simulink model "Lab4"  (R2023a)
settings: Solver=VariableStepAuto  StartTime=0.0  StopTime=20  RelTol=1e-3
settings Model: Creator=Lenovo  LastModifiedBy=Lenovo

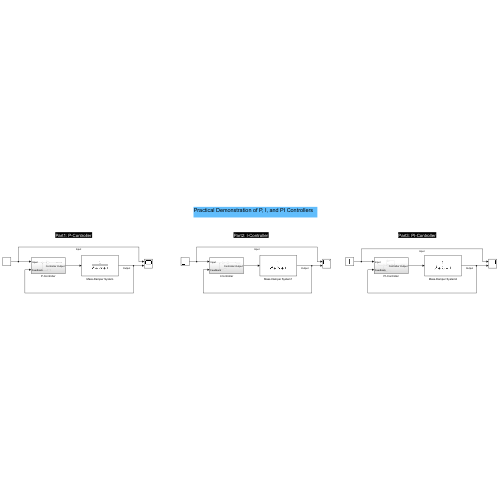
[thumbnail: Simulink's stored preview of the top-level diagram]
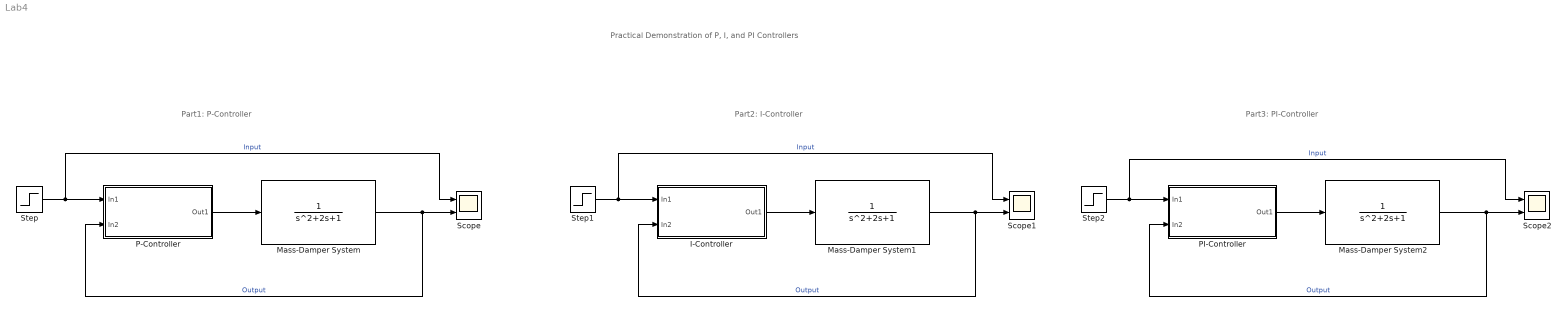
== system Lab4 ==
  note: Practical Demonstration of P, I, and PI Controllers
  note: Part1: P-Controller
  note: Part2: I-Controller
  note: Part3: PI-Controller
  I-Controller : Subsystem
  Mass-Damper System : TransferFcn
  Mass-Damper System1 : TransferFcn
  Mass-Damper System2 : TransferFcn
  P-Controller : Subsystem
  PI-Controller : Subsystem
  Scope : Scope  NumInputPorts=2
  Scope1 : Scope  NumInputPorts=2
  Scope2 : Scope  NumInputPorts=2
  Step : Step  SampleTime=0
  Step1 : Step  SampleTime=0
  Step2 : Step  SampleTime=0
  wires:
  Mass-Damper System/1 -> P-Controller/2(In2), Scope/2  "Output"
  Step/1 -> Scope/1, P-Controller/1(In1)  "Input"
  P-Controller/1(Out1) -> Mass-Damper System/1
  Mass-Damper System1/1 -> I-Controller/2(In2), Scope1/2  "Output"
  I-Controller/1(Out1) -> Mass-Damper System1/1
  Step1/1 -> Scope1/1, I-Controller/1(In1)  "Input"
  Step2/1 -> Scope2/1, PI-Controller/1(In1)  "Input"
  PI-Controller/1(Out1) -> Mass-Damper System2/1
  Mass-Damper System2/1 -> PI-Controller/2(In2), Scope2/2  "Output"

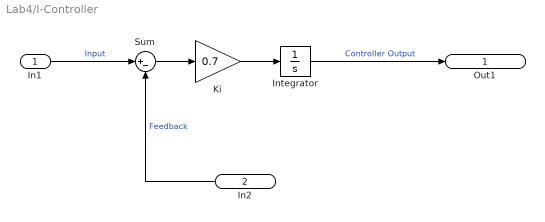
== system Lab4/I-Controller ==
  In1 : Inport
  In2 : Inport  Port=2
  Integrator : Integrator
  Ki : Gain  Gain=0.7
  Sum : Sum  Inputs=|+-
  Out1 : Outport
  wires:
  In1/1 -> Sum/1  "Input"
  Sum/1 -> Ki/1
  Ki/1 -> Integrator/1
  In2/1 -> Sum/2  "Feedback"
  Integrator/1 -> Out1/1  "Controller Output"

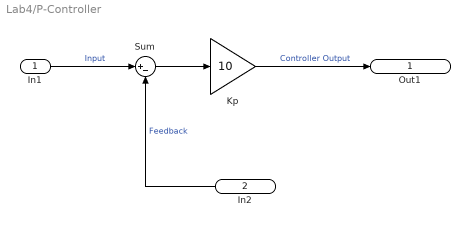
== system Lab4/P-Controller ==
  In1 : Inport
  In2 : Inport  Port=2
  Kp : Gain  Gain=10
  Sum : Sum  Inputs=|+-
  Out1 : Outport
  wires:
  In1/1 -> Sum/1  "Input"
  Sum/1 -> Kp/1
  Kp/1 -> Out1/1  "Controller Output"
  In2/1 -> Sum/2  "Feedback"

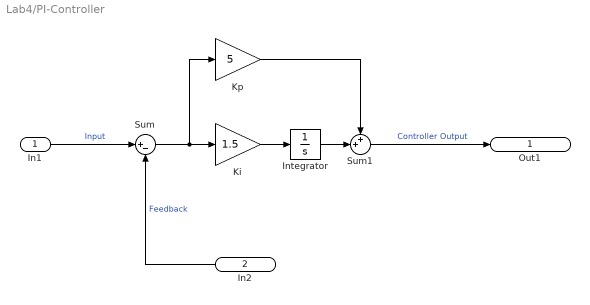
== system Lab4/PI-Controller ==
  In1 : Inport
  In2 : Inport  Port=2
  Integrator : Integrator
  Ki : Gain  Gain=1.5
  Kp : Gain  Gain=5
  Sum : Sum  Inputs=|+-
  Sum1 : Sum  Inputs=++|
  Out1 : Outport
  wires:
  In1/1 -> Sum/1  "Input"
  Sum/1 -> Kp/1, Ki/1
  Ki/1 -> Integrator/1
  In2/1 -> Sum/2  "Feedback"
  Integrator/1 -> Sum1/2
  Sum1/1 -> Out1/1  "Controller Output"
  Kp/1 -> Sum1/1
